simulink model "untitled"  (R2020a)
settings: Solver=VariableStepAuto  StartTime=0.0  StopTime=10.0  MaxStep=1e-3  RelTol=1e-3
undefined symbols (not defined in the file): g, l
settings Model: Creator=Marwan Mohamed  LastModifiedBy=Marwan Mohamed

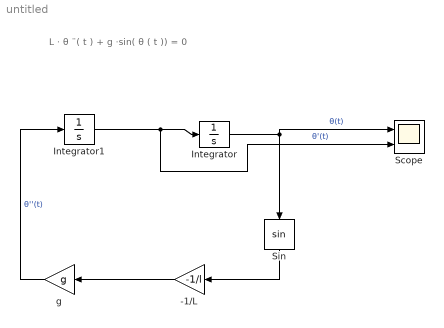
== system untitled ==
  note: L ⋅ θ ¨( t ) + g ⋅sin( θ ( t )) = 0
  -1/L : Gain  Gain=-1/l
  Integrator : Integrator  InitialCondition=1
  Integrator1 : Integrator
  Scope : Scope  NumInputPorts=2
  Sin : Trigonometry
  g : Gain  Gain=g
  wires:
  Sin/1 -> -1/L/1
  -1/L/1 -> g/1
  g/1 -> Integrator1/1  "θ''(t)"
  Integrator1/1 -> Scope/2, Integrator/1  "θ'(t)"
  Integrator/1 -> Sin/1, Scope/1  "θ(t)"
